simulink model "FullBridge_ModifiedUnipolarModulation"  (R2021b)
settings: Solver=FixedStepDiscrete  StartTime=0.0  StopTime=0.5  RelTol=1e-3
libraries: spsMosfetLib x4, spsSeriesRLCBranchLib x3, spsTriangleGeneratorLib x2, spsVoltageMeasurementLib x2, spsCurrentMeasurementLib x1, spsDCVoltageSourceLib x1, spspowerguiLib x1
settings Model: Creator=ycay  LastModifiedBy=ycay

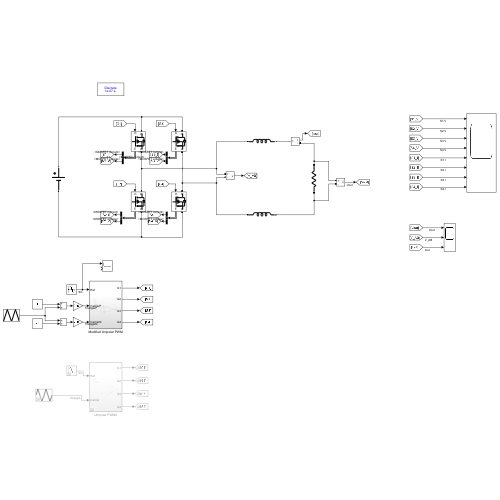
[thumbnail: Simulink's stored preview of the top-level diagram]
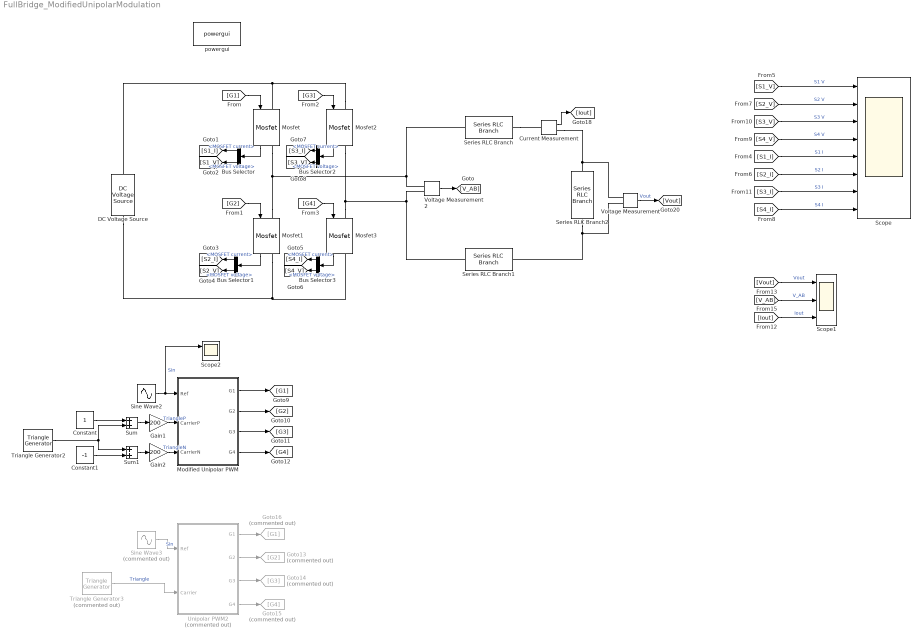
== system FullBridge_ModifiedUnipolarModulation ==
  Bus Selector{,1..3} (4 alike) : BusSelector  OutputSignals=MOSFET current,MOSFET voltage
  Constant : Constant
  Constant1 : Constant  Value=-1
  Current Measurement : spsCurrentMeasurementLib/Current Measurement  PhasorSimulation=off  OutputType=Complex  PSBequivalent=0
  DC Voltage Source : spsDCVoltageSourceLib/DC Voltage Source  Amplitude=400  Measurements=None
  Gain1 : Gain  Gain=200
  Gain2 : Gain  Gain=200
  Goto13 : Goto  Commented=on  GotoTag=G2
  Goto14 : Goto  Commented=on  GotoTag=G3
  Goto15 : Goto  Commented=on  GotoTag=G4
  Goto16 : Goto  Commented=on  GotoTag=G1
  Modified Unipolar PWM : Subsystem
  Mosfet{,1..3} (4 alike) : spsMosfetLib/Mosfet  Ron=0.001  Lon=0  Rd=0.001  Vfd=0  IC=0  Rs=1e5  Cs=inf  Measurements=on
  Scope : Scope  NumInputPorts=8
  Scope1 : Scope  NumInputPorts=3
  Scope2 : Scope  NumInputPorts=2
  Series RLC Branch : spsSeriesRLCBranchLib/Series RLC Branch  LConnTagsString=__new0  RConnTagsString=__new0  BranchType=L  Resistance=1  Inductance=10e-3  SetiL0=off  InitialCurrent=0  Capacitance=1e-6  Setx0=off  InitialVoltage=0  Measurements=None
  Series RLC Branch1 : spsSeriesRLCBranchLib/Series RLC Branch  LConnTagsString=__new0  RConnTagsString=__new0  BranchType=L  Resistance=1  Inductance=10e-3  SetiL0=off  InitialCurrent=0  Capacitance=1e-6  Setx0=off  InitialVoltage=0  Measurements=None
  Series RLC Branch2 : spsSeriesRLCBranchLib/Series RLC Branch  LConnTagsString=__new0  RConnTagsString=__new0  BranchType=R  Resistance=100  Inductance=1e-3  SetiL0=off  InitialCurrent=0  Capacitance=1e-6  Setx0=off  InitialVoltage=0  Measurements=None
  Sine Wave2 : Sin  Amplitude=325  Frequency=2*pi*50  Phase=pi/3  SampleTime=1e-6
  Sine Wave3 : Sin  Commented=on  Amplitude=325  Frequency=2*pi*50  SampleTime=1e-6
  Sum : Sum
  Sum1 : Sum
  Triangle Generator2 : spsTriangleGeneratorLib/Triangle Generator  Freq=1e5  Phase=0  Ts=1e-7
  Triangle Generator3 : spsTriangleGeneratorLib/Triangle Generator  Commented=on  Freq=1e5  Phase=90  Ts=1e-7
  Unipolar PWM2 : Subsystem  Commented=on
  Voltage Measurement : spsVoltageMeasurementLib/Voltage Measurement  PhasorSimulation=off  OutputType=Complex  PSBequivalent=0
  Voltage Measurement2 : spsVoltageMeasurementLib/Voltage Measurement  PhasorSimulation=off  OutputType=Complex  PSBequivalent=0
  powergui : spspowerguiLib/powergui  Priority=1  SimulationMode=Discrete  SampleTime=1e-7  frequency=60  Iterations=50  frequencyindice=0  Pbase=100e6  ErrMax=1e-4  UnitsV=kV  UnitsW=MW  buscounter=0  FunctionMessages=off  echomessages=off  EnableUseOfTLC=off  CurrentSourceSwitches=off  DisableSnubberDevices=off  DisableRonSwitches=off  DisableVfSwitches=off  DisplayEquations=off  AutomaticDiscreteSolvers=off  SolverType=Tustin/Backward Euler (TBE)  Interpol=off  ExternalGateDelay=off  methode=off  Ts=100  x0status=blocks  SPID=on  SwTol=0  HookPort=off  NonlinearTolerance=1e-4  nMaxIteration=100  ContinueOnMaxIteration=off  RestoreLinks=warning  ResistiveCurrentMeasurement=off  Frange=[0:2:500]  Ylog=off  Xlog=on  ShowGrid=off  save=off  variable=ZData  structure=0  ZoomFFT=off  StartTime=0.0  cycles=1  DisplayStyle=1  fundamental=60  FreqAxis=off  MaxFrequency=1000  frequencyindicesteady=1  RmsSteady=1  display=off
  wires:
  Bus Selector2/1 -> [S3_I]  "<MOSFET current>"
  Bus Selector2/2 -> [S3_V]  "<MOSFET voltage>"
  [G3] -> Mosfet2/1
  Voltage Measurement/1 -> [Vout]  "Vout"
  Current Measurement/1 -> [Iout]
  [G1] -> Mosfet/1
  Voltage Measurement2/1 -> [V_AB]
  Bus Selector3/2 -> [S4_V]  "<MOSFET voltage>"
  [G4] -> Mosfet3/1
  Bus Selector3/1 -> [S4_I]  "<MOSFET current>"
  Mosfet3/1 -> Bus Selector3/1
  Mosfet2/1 -> Bus Selector2/1
  Bus Selector1/1 -> [S2_I]  "<MOSFET current>"
  Mosfet/1 -> Bus Selector/1
  Bus Selector/2 -> [S1_V]  "<MOSFET voltage>"
  [S1_I] -> Scope/5  "S1 I"
  [S3_V] -> Scope/3  "S3 V"
  [Iout] -> Scope1/3  "Iout"
  [G2] -> Mosfet1/1
  [S3_I] -> Scope/7  "S3 I"
  [S4_I] -> Scope/8  "S4 I"
  [S1_V] -> Scope/1  "S1 V"
  Bus Selector/1 -> [S1_I]  "<MOSFET current>"
  [S2_V] -> Scope/2  "S2 V"
  [S2_I] -> Scope/6  "S2 I"
  [S4_V] -> Scope/4  "S4 V"
  [V_AB] -> Scope1/2  "V_AB"
  Bus Selector1/2 -> [S2_V]  "<MOSFET voltage>"
  Mosfet1/1 -> Bus Selector1/1
  [Vout] -> Scope1/1  "Vout"
  Modified Unipolar PWM/2(G2) -> [G2]
  Modified Unipolar PWM/4(G4) -> [G4]
  Modified Unipolar PWM/1(G1) -> [G1]
  Modified Unipolar PWM/3(G3) -> [G3]
  Sine Wave2/1 -> Scope2/1, Modified Unipolar PWM/1(Ref)  "Sin"
  Unipolar PWM2/4(G4) -> Goto15/1
  Triangle Generator3/1 -> Unipolar PWM2/2(Carrier)  "Triangle"
  Unipolar PWM2/1(G1) -> Goto16/1
  Sine Wave3/1 -> Unipolar PWM2/1(Ref)  "Sin"
  Unipolar PWM2/2(G2) -> Goto13/1
  Unipolar PWM2/3(G3) -> Goto14/1
  Sum/1 -> Gain1/1
  Triangle Generator2/1 -> Sum/2, Sum1/1
  Constant/1 -> Sum/1
  Sum1/1 -> Gain2/1
  Constant1/1 -> Sum1/2
  Gain2/1 -> Modified Unipolar PWM/3(CarrierN)  "TriangleN"
  Gain1/1 -> Modified Unipolar PWM/2(CarrierP)  "TriangleP"
  connections:
  Series RLC Branch2/LConn1 -- Current Measurement/RConn1 -- Voltage Measurement/LConn1
  Mosfet1/LConn1 -- Mosfet/RConn1 -- Voltage Measurement2/LConn1 -- Series RLC Branch/LConn1
  Mosfet2/LConn1 -- Mosfet/LConn1 -- DC Voltage Source/RConn1
  Mosfet3/LConn1 -- Mosfet2/RConn1 -- Voltage Measurement2/LConn2 -- Series RLC Branch1/RConn1
  Voltage Measurement/LConn2 -- Series RLC Branch2/RConn1 -- Series RLC Branch1/LConn1
  Mosfet3/RConn1 -- DC Voltage Source/LConn1 -- Mosfet1/RConn1
  Series RLC Branch/RConn1 -- Current Measurement/LConn1

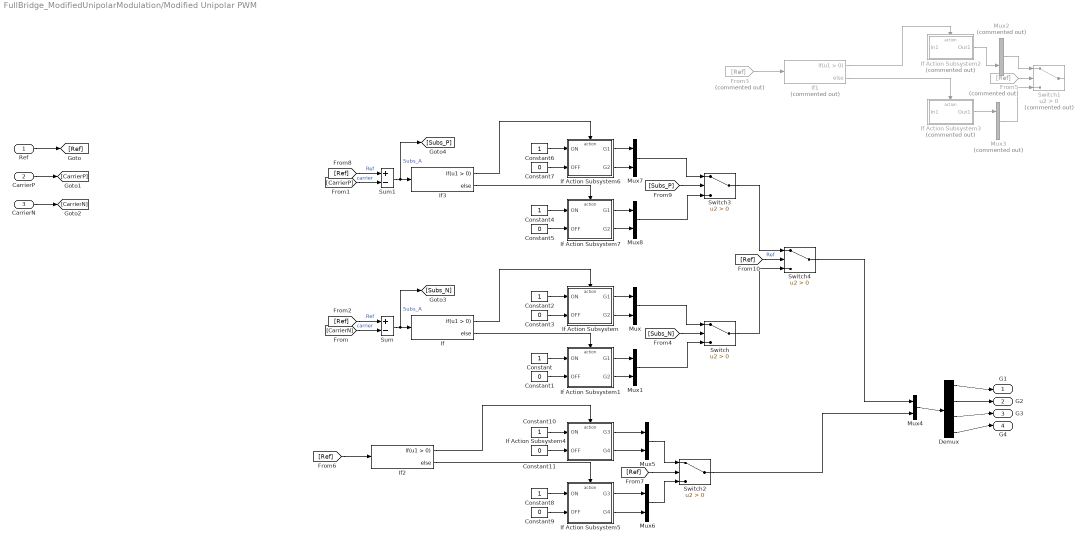
== system FullBridge_ModifiedUnipolarModulation/Modified Unipolar PWM ==
  Ref : Inport
  CarrierP : Inport  Port=2
  CarrierN : Inport  Port=3
  Constant{,2,4,6,8,10} (6 alike) : Constant
  Constant{1,3,5,7,9,11} (6 alike) : Constant  Value=0
  Demux : Demux
  From3 : From  Commented=on  GotoTag=Ref
  From5 : From  Commented=on  GotoTag=Ref
  If : If
  If Action Subsystem : Subsystem  TreatAsAtomicUnit=on
  If Action Subsystem1 : Subsystem  TreatAsAtomicUnit=on
  If Action Subsystem2 : Subsystem  Commented=on  TreatAsAtomicUnit=on
  If Action Subsystem3 : Subsystem  Commented=on  TreatAsAtomicUnit=on
  If Action Subsystem4 : Subsystem  TreatAsAtomicUnit=on
  If Action Subsystem5 : Subsystem  TreatAsAtomicUnit=on
  If Action Subsystem6 : Subsystem  TreatAsAtomicUnit=on
  If Action Subsystem7 : Subsystem  TreatAsAtomicUnit=on
  If1 : If  Commented=on
  If2 : If
  If3 : If
  Mux{,1,4..8} (7 alike) : Mux  Inputs=2
  Mux2 : Mux  Commented=on  Inputs=2
  Mux3 : Mux  Commented=on  Inputs=2
  Sum : Sum  Inputs=+-
  Sum1 : Sum  Inputs=+-
  Switch{,2..4} (4 alike) : Switch  Criteria=u2 > Threshold
  Switch1 : Switch  Commented=on  Criteria=u2 > Threshold
  G1 : Outport
  G2 : Outport  Port=2
  G3 : Outport  Port=3
  G4 : Outport  Port=4
  wires:
  Demux/4 -> G4/1
  Demux/3 -> G3/1
  Mux4/1 -> Demux/1
  Mux1/1 -> Switch/3
  Mux/1 -> Switch/1
  [Subs_N] -> Switch/2
  Sum/1 -> If/1, [Subs_N]  "Subs_A"
  Constant2/1 -> If Action Subsystem/1(ON)
  If Action Subsystem1/1(G1) -> Mux1/1
  If Action Subsystem1/2(G2) -> Mux1/2
  Constant3/1 -> If Action Subsystem/2(OFF)
  Constant/1 -> If Action Subsystem1/1(ON)
  If Action Subsystem/2(G2) -> Mux/2
  If Action Subsystem/1(G1) -> Mux/1
  If/2 -> If Action Subsystem1/Action
  If/1 -> If Action Subsystem/Action
  Constant1/1 -> If Action Subsystem1/2(OFF)
  [CarrierN] -> Sum/2  "carrier"
  [Ref] -> Sum/1  "Ref"
  Demux/2 -> G2/1
  Demux/1 -> G1/1
  [Ref] -> If2/1
  Constant10/1 -> If Action Subsystem4/1(ON)
  Constant11/1 -> If Action Subsystem4/2(OFF)
  Constant8/1 -> If Action Subsystem5/1(ON)
  If2/2 -> If Action Subsystem5/Action
  If2/1 -> If Action Subsystem4/Action
  Constant9/1 -> If Action Subsystem5/2(OFF)
  [Ref] -> Switch2/2
  If Action Subsystem4/2(G4) -> Mux5/2
  If Action Subsystem4/1(G3) -> Mux5/1
  Mux5/1 -> Switch2/1
  If Action Subsystem5/1(G3) -> Mux6/1
  If Action Subsystem5/2(G4) -> Mux6/2
  Mux6/1 -> Switch2/3
  Switch2/1 -> Mux4/2
  From3/1 -> If1/1
  If1/1 -> If Action Subsystem2/Action
  If1/2 -> If Action Subsystem3/Action
  If Action Subsystem2/1(Out1) -> Mux2/2
  Mux2/1 -> Switch1/1
  If Action Subsystem3/1(Out1) -> Mux3/1
  Mux3/1 -> Switch1/3
  From5/1 -> Switch1/2
  CarrierN/1 -> [CarrierN]
  CarrierP/1 -> [CarrierP]
  Ref/1 -> [Ref]
  [Ref] -> Sum1/1  "Ref"
  [CarrierP] -> Sum1/2  "carrier"
  Constant5/1 -> If Action Subsystem7/2(OFF)
  If3/1 -> If Action Subsystem6/Action
  If3/2 -> If Action Subsystem7/Action
  If Action Subsystem6/1(G1) -> Mux7/1
  If Action Subsystem6/2(G2) -> Mux7/2
  Constant4/1 -> If Action Subsystem7/1(ON)
  Constant7/1 -> If Action Subsystem6/2(OFF)
  If Action Subsystem7/2(G2) -> Mux8/2
  If Action Subsystem7/1(G1) -> Mux8/1
  Constant6/1 -> If Action Subsystem6/1(ON)
  Sum1/1 -> [Subs_P], If3/1  "Subs_A"
  [Subs_P] -> Switch3/2
  Mux7/1 -> Switch3/1
  Mux8/1 -> Switch3/3
  Switch3/1 -> Switch4/1
  Switch/1 -> Switch4/3
  [Ref] -> Switch4/2  "Ref"
  Switch4/1 -> Mux4/1

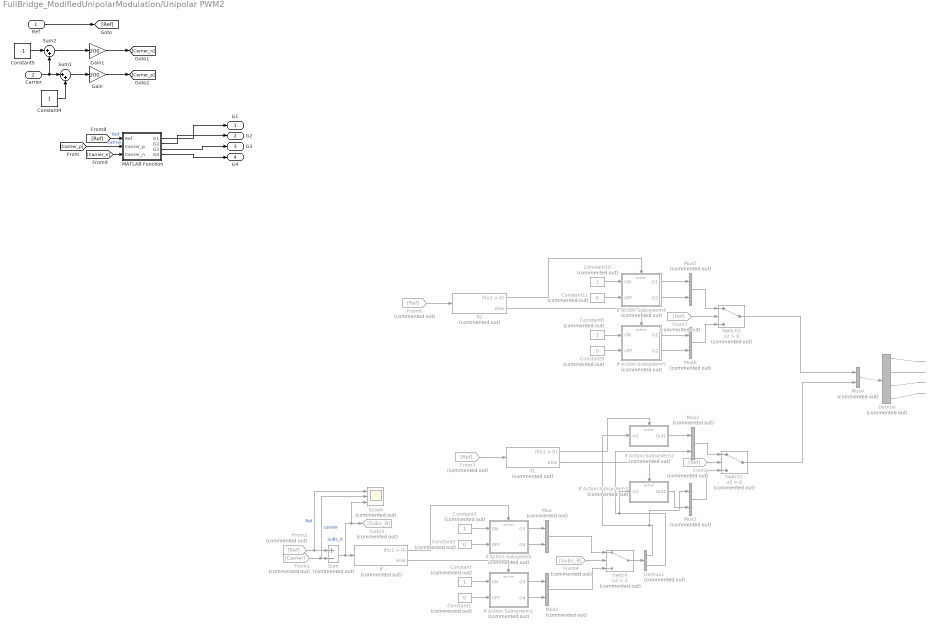
== system FullBridge_ModifiedUnipolarModulation/Unipolar PWM2 ==
  Ref : Inport
  Carrier : Inport  Port=2
  Constant{,2,8,10} (4 alike) : Constant  Commented=on
  Constant{1,3,9,11} (4 alike) : Constant  Commented=on  Value=0
  Constant4 : Constant
  Constant5 : Constant  Value=-1
  Demux : Demux  Commented=on
  Demux1 : Demux  Commented=on  Outputs=2
  From1 : From  Commented=on  GotoTag=Carrier
  From{2..3,5..7} (5 alike) : From  Commented=on  GotoTag=Ref
  From4 : From  Commented=on  GotoTag=Subs_B
  Gain : Gain  Gain=200
  Gain1 : Gain  Gain=200
  Goto3 : Goto  Commented=on  GotoTag=Subs_B
  If : If  Commented=on
  If Action Subsystem : Subsystem  Commented=on  TreatAsAtomicUnit=on
  If Action Subsystem1 : Subsystem  Commented=on  TreatAsAtomicUnit=on
  If Action Subsystem2 : Subsystem  Commented=on  TreatAsAtomicUnit=on
  If Action Subsystem3 : Subsystem  Commented=on  TreatAsAtomicUnit=on
  If Action Subsystem4 : Subsystem  Commented=on  TreatAsAtomicUnit=on
  If Action Subsystem5 : Subsystem  Commented=on  TreatAsAtomicUnit=on
  If1 : If  Commented=on
  If2 : If  Commented=on
  MATLAB Function : MATLAB Function  TreatAsAtomicUnit=on
  Mux{,1..6} (7 alike) : Mux  Commented=on  Inputs=2
  Scope : Scope  Commented=on  NumInputPorts=3
  Sum : Sum  Commented=on  Inputs=+-
  Sum1 : Sum  Inputs=|++
  Sum2 : Sum  Inputs=|++
  Switch : Switch  Commented=on  Criteria=u2 > Threshold
  Switch1 : Switch  Commented=on  Criteria=u2 > Threshold
  Switch2 : Switch  Commented=on  Criteria=u2 > Threshold
  G1 : Outport
  G2 : Outport  Port=2
  G3 : Outport  Port=3
  G4 : Outport  Port=4
  wires:
  From5/1 -> Switch1/2
  Mux3/1 -> Switch1/3
  Mux2/1 -> Switch1/1
  Switch/1 -> Demux1/1
  If1/2 -> If Action Subsystem3/Action
  If1/1 -> If Action Subsystem2/Action
  From3/1 -> If1/1
  Mux6/1 -> Switch2/3
  If Action Subsystem5/2(G2) -> Mux6/2
  If Action Subsystem5/1(G1) -> Mux6/1
  Mux5/1 -> Switch2/1
  If Action Subsystem4/1(G1) -> Mux5/1
  If Action Subsystem4/2(G2) -> Mux5/2
  From7/1 -> Switch2/2
  Constant9/1 -> If Action Subsystem5/2(OFF)
  If2/1 -> If Action Subsystem4/Action
  If2/2 -> If Action Subsystem5/Action
  Constant8/1 -> If Action Subsystem5/1(ON)
  Constant11/1 -> If Action Subsystem4/2(OFF)
  Constant10/1 -> If Action Subsystem4/1(ON)
  From6/1 -> If2/1
  Demux/1 -> ?
  Demux/2 -> ?
  Ref/1 -> [Ref]
  From2/1 -> Sum/1, Scope/1  "Ref"
  From1/1 -> Sum/2, Scope/2  "carrier"
  Constant1/1 -> If Action Subsystem1/2(OFF)
  If/1 -> If Action Subsystem/Action
  If/2 -> If Action Subsystem1/Action
  If Action Subsystem/1(G3) -> Mux/1
  If Action Subsystem/2(G4) -> Mux/2
  Constant/1 -> If Action Subsystem1/1(ON)
  Constant3/1 -> If Action Subsystem/2(OFF)
  If Action Subsystem1/2(G4) -> Mux1/2
  If Action Subsystem1/1(G3) -> Mux1/1
  Constant2/1 -> If Action Subsystem/1(ON)
  Sum/1 -> Goto3/1, Scope/3, If/1  "Subs_A"
  From4/1 -> Switch/2
  Mux/1 -> Switch/1
  Mux1/1 -> Switch/3
  Mux4/1 -> Demux/1
  Demux/3 -> ?
  Demux/4 -> ?
  Switch2/1 -> Mux4/1
  Switch1/1 -> Mux4/2
  Demux1/1 -> Mux3/1, If Action Subsystem2/1(In1)
  Demux1/2 -> Mux2/2, If Action Subsystem3/1(In1)
  If Action Subsystem3/1(Out1) -> Mux3/2
  If Action Subsystem2/1(Out1) -> Mux2/1
  [Ref] -> MATLAB Function/1(Ref)  "Ref"
  [Carrier_p] -> MATLAB Function/2(Carrier_p)  "carrier"
  MATLAB Function/1(G1) -> G1/1
  MATLAB Function/2(G2) -> G2/1
  MATLAB Function/3(G3) -> G3/1
  MATLAB Function/4(G4) -> G4/1
  Carrier/1 -> Sum2/2, Sum1/1
  Constant4/1 -> Sum1/2
  Sum1/1 -> Gain/1
  Gain/1 -> [Carrier_p]
  Constant5/1 -> Sum2/1
  Sum2/1 -> Gain1/1
  Gain1/1 -> [Carrier_n]
  [Carrier_n] -> MATLAB Function/3(Carrier_n)

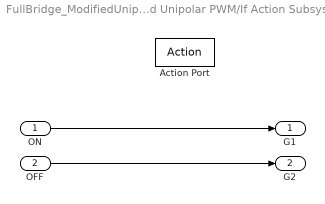
== system FullBridge_ModifiedUnipolarModulation/Modified Unipolar PWM/If Action Subsystem ==
  ON : Inport
  OFF : Inport  Port=2
  Action Port : ActionPort  ActionPortLabel=if(u1 > 0)
  G1 : Outport
  G2 : Outport  Port=2
  wires:
  OFF/1 -> G2/1
  ON/1 -> G1/1

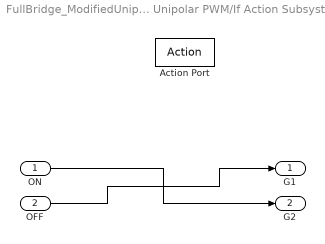
== system FullBridge_ModifiedUnipolarModulation/Modified Unipolar PWM/If Action Subsystem1 ==
  ON : Inport
  OFF : Inport  Port=2
  Action Port : ActionPort  ActionPortLabel=else
  G1 : Outport
  G2 : Outport  Port=2
  wires:
  OFF/1 -> G1/1
  ON/1 -> G2/1

== system FullBridge_ModifiedUnipolarModulation/Modified Unipolar PWM/If Action Subsystem2 ==
  In1 : Inport
  Action Port : ActionPort  ActionPortLabel=if(u1 > 0)
  Gain : Gain  Gain=0
  Out1 : Outport
  wires:
  In1/1 -> Gain/1
  Gain/1 -> Out1/1

== system FullBridge_ModifiedUnipolarModulation/Modified Unipolar PWM/If Action Subsystem3 ==
  In1 : Inport
  Action Port : ActionPort  ActionPortLabel=else
  Gain : Gain  Gain=0
  Out1 : Outport
  wires:
  In1/1 -> Gain/1
  Gain/1 -> Out1/1

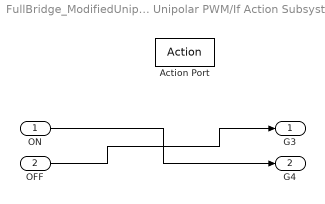
== system FullBridge_ModifiedUnipolarModulation/Modified Unipolar PWM/If Action Subsystem4 ==
  ON : Inport
  OFF : Inport  Port=2
  Action Port : ActionPort  ActionPortLabel=if(u1 > 0)
  G3 : Outport
  G4 : Outport  Port=2
  wires:
  ON/1 -> G4/1
  OFF/1 -> G3/1

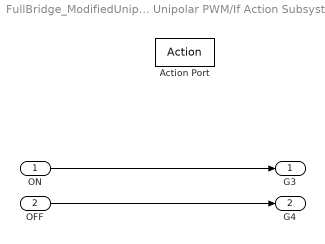
== system FullBridge_ModifiedUnipolarModulation/Modified Unipolar PWM/If Action Subsystem5 ==
  ON : Inport
  OFF : Inport  Port=2
  Action Port : ActionPort  ActionPortLabel=else
  G3 : Outport
  G4 : Outport  Port=2
  wires:
  ON/1 -> G3/1
  OFF/1 -> G4/1

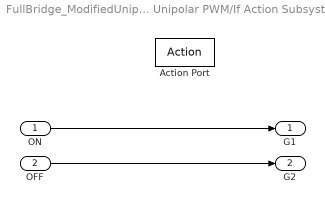
== system FullBridge_ModifiedUnipolarModulation/Modified Unipolar PWM/If Action Subsystem6 ==
  ON : Inport
  OFF : Inport  Port=2
  Action Port : ActionPort  ActionPortLabel=if(u1 > 0)
  G1 : Outport
  G2 : Outport  Port=2
  wires:
  ON/1 -> G1/1
  OFF/1 -> G2/1

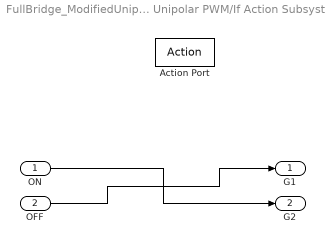
== system FullBridge_ModifiedUnipolarModulation/Modified Unipolar PWM/If Action Subsystem7 ==
  ON : Inport
  OFF : Inport  Port=2
  Action Port : ActionPort  ActionPortLabel=else
  G1 : Outport
  G2 : Outport  Port=2
  wires:
  ON/1 -> G2/1
  OFF/1 -> G1/1

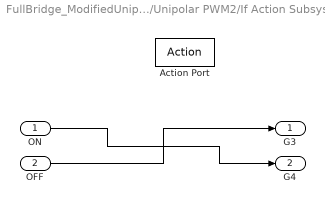
== system FullBridge_ModifiedUnipolarModulation/Unipolar PWM2/If Action Subsystem ==
  ON : Inport
  OFF : Inport  Port=2
  Action Port : ActionPort
  G3 : Outport
  G4 : Outport  Port=2
  wires:
  OFF/1 -> G3/1
  ON/1 -> G4/1

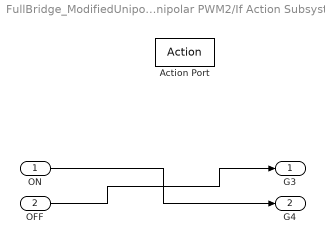
== system FullBridge_ModifiedUnipolarModulation/Unipolar PWM2/If Action Subsystem1 ==
  ON : Inport
  OFF : Inport  Port=2
  Action Port : ActionPort
  G3 : Outport
  G4 : Outport  Port=2
  wires:
  ON/1 -> G4/1
  OFF/1 -> G3/1

== system FullBridge_ModifiedUnipolarModulation/Unipolar PWM2/If Action Subsystem2 ==
  In1 : Inport
  Action Port : ActionPort
  Gain : Gain  Gain=0
  Out1 : Outport
  wires:
  Gain/1 -> Out1/1
  In1/1 -> Gain/1

== system FullBridge_ModifiedUnipolarModulation/Unipolar PWM2/If Action Subsystem3 ==
  In1 : Inport
  Action Port : ActionPort
  Gain : Gain  Gain=0
  Out1 : Outport
  wires:
  Gain/1 -> Out1/1
  In1/1 -> Gain/1

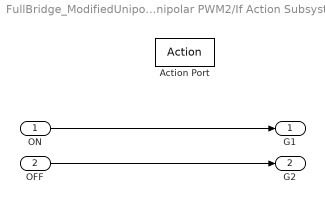
== system FullBridge_ModifiedUnipolarModulation/Unipolar PWM2/If Action Subsystem4 ==
  ON : Inport
  OFF : Inport  Port=2
  Action Port : ActionPort
  G1 : Outport
  G2 : Outport  Port=2
  wires:
  ON/1 -> G1/1
  OFF/1 -> G2/1

== system FullBridge_ModifiedUnipolarModulation/Unipolar PWM2/If Action Subsystem5 ==
  ON : Inport
  OFF : Inport  Port=2
  Action Port : ActionPort
  G1 : Outport
  G2 : Outport  Port=2
  wires:
  OFF/1 -> G1/1
  ON/1 -> G2/1

== matlab function FullBridge_ModifiedUnipolarModulation/Unipolar PWM2/MATLAB Function ==
  data: Ref input; G1 output; Carrier_p input; G2 output; G3 output; G4 output; Carrier_n input
function [G1,G2,G3,G4] = fcn(Ref,Carrier_p,Carrier_n)
Subs_B_p = Ref - Carrier_p;
Subs_B_n = Ref - Carrier_n;
if (Ref > 0)
    G1 = 1;
    G2 = 0;
    if (Subs_B_p > 0)
        G3 = 0;
        G4 = 1;
    else
        G3 = 0;
        G4 = 0;
    end
else
    G1 = 0;
    G2 = 1;
    if (Subs_B_n < 0)
        G3 = 1;
        G4 = 0;
    else
        G3 = 0;
        G4 = 0;
    end
end
